simulink model "AmbientSIL_TestBed"  (R2016b)
settings: Solver=FixedStepDiscrete  StartTime=0.0  StopTime=1  FixedStep=1  RelTol=1e-3  EnableMultiTasking=on
undefined symbols (not defined in the file): MWS
settings Model: Creator=jwchapm2  LastModifiedBy=jwchapm2
settings DataIOCC: LimitDataPoints=on  SaveFormat=Array
settings OptimizationCC: DefaultParameterBehavior=Inlined  ExpressionDepthLimit=2147483647
settings DebuggingCC: UnderspecifiedInitializationDetection=Classic  MergeDetectMultiDrivingBlocksExec=none  SolverPrmCheckMsg=warning  ParameterTunabilityLossMsg=error  StateNameClashWarn=warning  SFUnexpectedBacktrackingDiag=warning  SFNoUnconditionalDefaultTransitionDiag=warning  SFExecutionAtInitializationDiag=none
settings HardwareCC: ProdBitPerPointer=32  ProdBitPerSizeT=32  ProdBitPerPtrDiffT=32  ProdLargestAtomicFloat=None  ProdIntDivRoundTo=Undefined  ProdEndianess=Unspecified  ProdWordSize=32  ProdHWDeviceType=32-bit Generic
settings ModelReferenceCC: PropagateSignalLabelsOutOfModel=off
settings RTWCC: SystemTargetFile=ert.tlc  TemplateMakefile=ert_default_tmf  Description=Embedded Coder  GenerateReport=on  IncludeHyperlinkInReport=on  LaunchReport=on  GenerateTraceInfo=on  GenerateTraceReport=on  GenerateTraceReportSl=on  GenerateTraceReportSf=on  GenerateTraceReportEml=on
settings CodeAppCC: ForceParamTrailComments=on  IgnoreCustomStorageClasses=off  OperatorAnnotations=on  SimulinkDataObjDesc=on  SFDataObjDesc=on  MATLABFcnDesc=on  InsertBlockDesc=on  MATLABSourceComments=on
settings ERTTargetCC: GenerateSampleERTMain=on  InlinedParameterPlacement=NonHierarchical  ERTCustomFileTemplate=example_file_process.tlc
settings ConfigComp: CovMetricSettings=dw  CovHtmlReporting=on  CovSaveCumulativeToWorkspaceVar=on  CovSaveSingleToWorkspaceVar=on  CovExternalEMLEnable=off

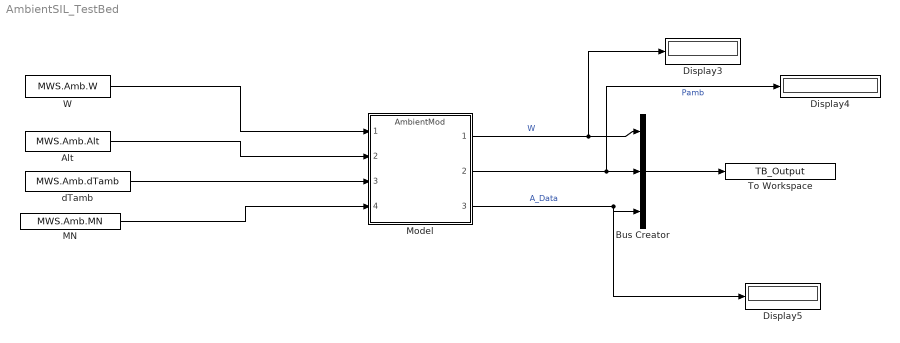
== system AmbientSIL_TestBed ==
  Alt : Constant  Value=MWS.Amb.Alt
  Bus Creator : BusCreator  Inputs=3
  Display3 : Display
  Display4 : Display
  Display5 : Display
  MN : Constant  Value=MWS.Amb.MN
  Model : ModelReference  ModelNameDialog=AmbientMod.slx  SimulationMode=Software-in-the-loop (SIL)  ModelReferenceVersion=1.21
  To Workspace : ToWorkspace  VariableName=TB_Output  SampleTime=-1
  W : Constant  Value=MWS.Amb.W
  dTamb : Constant  Value=MWS.Amb.dTamb
  wires:
  W/1 -> Model/1
  dTamb/1 -> Model/3
  Model/1 -> Bus Creator/1, Display3/1  "W"
  Model/2 -> Bus Creator/2, Display4/1  "Pamb"
  Model/3 -> Display5/1, Bus Creator/3  "A_Data"
  Bus Creator/1 -> To Workspace/1
  MN/1 -> Model/4
  Alt/1 -> Model/2
